simulink model "Vcu"  (R2020a)
settings: Solver=FixedStepDiscrete  StartTime=0.0  StopTime=10.0  FixedStep=ModelSimTime  RelTol=1e-3
PostLoadFcn:
  | , if any(exist('dsrtsu_mdlpostloadfcn', 'file') ~= 0), dsrtsu_mdlpostloadfcn('Execute', bdroot); end,
InitFcn:
  | , if any(exist('rtifpga_mdlclblib', 'file') ~= 0), rtifpga_mdlclblib('Init', bdroot); end,
undefined symbols (not defined in the file): rticanmm_blockfcn, rticanmm_initfcn, sigbuilder_block
libraries: rtimmsu_dsrtlib x5, commutil2 x1
(part 2 of 3)

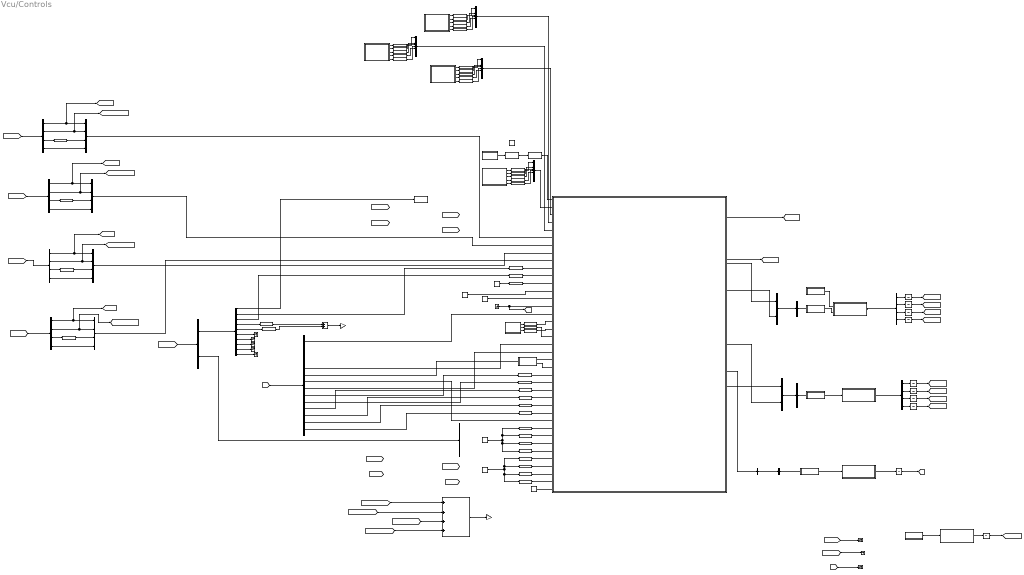
== system Vcu/Controls  ==
  Add : Sum  Inputs=++++
  Add1 : Sum  AccumDataTypeStr=double
  Bus Creator : BusCreator  Inputs=2
  Bus Creator1 : BusCreator  Inputs=2
  Bus Creator{7..10} (4 alike) : BusCreator  Inputs=11
  Bus Creator2 : BusCreator  Inputs=1
  Bus Creator{3..6} (4 alike) : BusCreator  Inputs=4  OutDataTypeStr=Bus: AmkActualValues2
  Bus Selector : BusSelector  OutputSignals=Inverter1FL,Inverter2FR  OutputAsBus=on
  Bus Selector1 : BusSelector  OutputSignals=AMK0_ActualValues1,AMK1_ActualValues1,AMK0_ActualValues2,AMK1_ActualValues2
  Bus Selector10 : BusSelector  OutputSignals=MotorLoopFluidTemp,InverterLoopFluidTemp,MotorLoopPressure,InverterLoopPressure
  Bus Selector11 : BusSelector  OutputSignals=ELP_StateInfo.ELP_BmsFault,ELP_StateInfo.ELP_ContactorK1,ELP_StateInfo.ELP_ContactorK2,ELP_StateInfo.ELP_ContactorK3,ELP_StateInfo.ELP_RelayFault,ELP_StateInfo.ELP_Flags_uint8,ELP_StateInfo.ELP_FltCodeStored_uint8,ELP_StateInfo.ELP_LevelFaultFlags,ELP_SOCInfo.ELP_SOC_pc,ELP_CurrentInfo.ELP_PackCurrent_A,ELP_CurrentInfo.ELP_ChargeCurrentMax_A,ELP_CurrentInfo.ELP_DischargeCurrentMax_A,ELP_VoltageInfo.ELP_PackVoltage_V,ELP_TemperatureInfo.ELP_PackAvgTemp_degC
  Bus Selector{4..6,12} (4 alike) : BusSelector  OutputSignals=AMK_TempMotor,AMK_TempInverter,AMK_ErrorInfo,AMK_TempIGBT
  Bus Selector2 : BusSelector  OutputSignals=AMK0_ActualValues1,AMK1_ActualValues1,AMK0_ActualValues2,AMK1_ActualValues2
  Bus Selector3 : BusSelector  OutputSignals=Inverter3RL,Inverter4RR  OutputAsBus=on
  Bus Selector7 : BusSelector  OutputSignals=contactor  OutputAsBus=on
  Bus Selector8 : BusSelector  OutputSignals=DriveButton,AcceleratorPedalPosition0,AcceleratorPedalPosition1,BrakePedalPosition0,BrakePedalPosition1,Apps0Status,Apps1Status,Bpps0Status,Bpps1Status,BspdFault
  Bus Selector9 : BusSelector  OutputSignals=PedalPositions,CoolingLoopsData
  Cast To Boolean{,1..22} (23 alike) : DataTypeConversion  OutDataTypeStr=boolean
  Constant : Constant
  Constant1 : Constant
  Constant2 : Constant  Value=20
  Constant3 : Constant  Value=20
  Constant4 : Constant  Value=20
  Constant6 : Constant  Value=100
  Constant7 : Constant  Value=0
  Data Type Conversion : DataTypeConversion  OutDataTypeStr=Enum: DRIVER_BUTTON
  Data Type Conversion{1..23} (23 alike) : DataTypeConversion  OutDataTypeStr=double
  Data Type Conversion24 : DataTypeConversion  OutDataTypeStr=Enum: DRIVER_BUTTON
  Data Type Conversion25 : DataTypeConversion  OutDataTypeStr=uint8
  Gain : Gain  Gain=1/4
  Gain1 : Gain  Gain=1/2  OutDataTypeStr=double
  Ground : Ground
  Model : ModelReference  ModelNameDialog=Controls.slx  SimulationMode=Normal  ModelReferenceVersion=1.57
  RTICANMM MainBlock : Subsystem  InitFcn=rticanmm_blockfcn('InitFcn', 'CANnedy', gcb)  ClipboardFcn=rticanmm_blockfcn('ClipboardFcn', 'CANnedy', gcb)  mask(RTICANMM){DSProperties=struct('RTI',struct('Version',uint32(1),'BlockType',struct('isSLSource',uint8(1),'isSLSink',uint8(1),'isHWSource',uint8(0),'isHWSink',uint8(0),'isSetup',uint8(0),'isInline',uint8(1),'isNonInline',uint8(0),'isInterrupt',uint8(0),'isChannelwise',uint8(0)),'IOBoardType','RTICANMM','UnitType','RTICANMM','Identifier','Mainblock','DialogType','SL','BlockSet','RTICANMM','SlaveProcessor','CAN')), CANMMProperties=struct('RTICANMMVersion','5.4','RTICANMMVersionIntern','5.4.737888.359837963','RTICANMMDate','02-May-2020','Settings','RTICANMM_MAIN_CAN_Amk1','UserTracePath','','ModelPath','C:\Users\harjo\Git\MACFormulaGit\MicroAutobox\microAutoboxModels\ControlsVcu','filesettings',struct('FileName','..\..\..\CAN_Databases\CAN_AMKInverter_1.dbc','IsRelative',1,'ClusterId',1,'ClusterList',{{'default'}},'destfolder',struct('Name','RTICANMM_FILES','Check',1),'buildfolder',struct('Name','.','Check',1),'onlyfreerawcapture',0,'overlapping2variant',0,'canfdsupport',0,'shortestJ2container',1),'onlyfreerawcapture',0,'Board',['CAN Type 1'],'BoardNum','1','ChannelNum','1','Variation','1','SetupId','Amk1','MARK',['30B141190671575CDE9C61D58C158C';'625D2D9E4FA6805ED198087D0F7A70';'291D995F13C69D1BB521FD81278AB5';'0D32706B1F9558B19EB16214799388';'2E4D033EB29162329D08EE38258F6F'],'date','08-Jul-2020','clock',['08.07.2020 00:50:18'],'recreate',0,'RTIVER','RTI1401','j1939',0,'TRC',struct('include',1),'rtsupport',struct('XMLFile','C:\Users\harjo\Git\MACFormulaGit\MicroAutobox\microAutoboxModels\ControlsVcu\RTICANMM_FILES\RTICANMM_MAIN_CAN_Amk1.xml','DBCXML',struct('Path','C:\Users\harjo\Git\MACFormulaGit\MicroAutobox\microAutoboxModels\ControlsVcu\RTICANMM_FILES\RTICANMM_MAIN_CAN_Amk1_dbc.xml','support',1,'Name','CAN_AMKInverter_1.dbc','Date',['23-Sep-2019 17:54:42'],'Type','standard','DBCSupport','ON'))), CANMMType=CANnedy, CANMMUserTraceMerged=off, CANMMUserTracePath=, CANMMChannelNum=1, CANMMBoardNum=1, CANMMDestFolder=RTICANMM_FILES, CANMMFolder=., CANMMSetupId=Amk1, CANMMsave2mat=['30B141190671575CDE9C61D58C158C';'625D2D9E4FA6805ED198087D0F7A70';'291D995F13C69D1BB521FD81278AB5';'0D32706B1F9558B19EB16214799388';'2E4D033EB29162329D08EE38258F6F'], CANMMName=CAN_Amk1, CANMMSettings=RTICANMM_MAIN_CAN_Amk1, CANMMIntermediateTag=RTICANMM_MAIN_CAN_Amk1_intermediate, CANMMsfcnname=RTICANMM_MAIN_CAN_Amk1}
      mask init:
      | rticanmm_initfcn(gcb, CANMMType, CANMMsfcnname)
      settings: AttributesFormatString=Amk1[CAN_Amk1]: DS1401_B1_C1_V1  CopyFcn=rticanmm_blockfcn('CopyFcn', 'CANnedy', gcb)  DeleteFcn=rticanmm_blockfcn('DeleteFcn', 'CANnedy', gcb)  ModelCloseFcn=rticanmm_blockfcn('ModelCloseFcn', 'CANnedy', gcb)  NameChangeFcn=rticanmm_blockfcn('NameChangeFcn', 'CANnedy', gcb)  OpenFcn=try, rticanmm_main_gui('create',gcb); ; catch,errordlg({lasterr, '','Please check your RTI installation.'},['Error: ' upper(bdroot)], 'replace'); end  MoveFcn=rticanmm_blockfcn('MoveFcn', 'CANnedy', gcb)
      mask Help: eval('rticanmm_quickstart(''create'', gcb);', 'disp(lasterr);')
      mask Display:
      | disp(sprintf('RTI CAN\nMultiMessage\nMainBlock'))
      | port_label('input', 1, 'Triggering')
      | port_label('input', 2, 'TX Data')
      | port_label('output', 1, 'RX Data')
  RTICANMM MainBlock1 : Subsystem  InitFcn=rticanmm_blockfcn('InitFcn', 'CANnedy', gcb)  ClipboardFcn=rticanmm_blockfcn('ClipboardFcn', 'CANnedy', gcb)  mask(RTICANMM){DSProperties=struct('RTI',struct('Version',uint32(1),'BlockType',struct('isSLSource',uint8(1),'isSLSink',uint8(1),'isHWSource',uint8(0),'isHWSink',uint8(0),'isSetup',uint8(0),'isInline',uint8(1),'isNonInline',uint8(0),'isInterrupt',uint8(0),'isChannelwise',uint8(0)),'IOBoardType','RTICANMM','UnitType','RTICANMM','Identifier','Mainblock','DialogType','SL','BlockSet','RTICANMM','SlaveProcessor','CAN')), CANMMProperties=struct('RTICANMMVersion','5.4','RTICANMMVersionIntern','5.4.737888.359837963','RTICANMMDate','02-May-2020','Settings','RTICANMM_MAIN_CAN_Amk2','UserTracePath','','ModelPath','C:\Users\harjo\Git\MACFormulaGit\MicroAutobox\microAutoboxModels\ControlsVcu','filesettings',struct('FileName','..\..\..\CAN_Databases\CAN_AMKInverter_2.dbc','IsRelative',1,'ClusterId',1,'ClusterList',{{'default'}},'destfolder',struct('Name','RTICANMM_FILES','Check',1),'buildfolder',struct('Name','.','Check',1),'onlyfreerawcapture',0,'overlapping2variant',0,'canfdsupport',0,'shortestJ2container',1),'onlyfreerawcapture',0,'Board',['CAN Type 1'],'BoardNum','1','ChannelNum','2','Variation','1','SetupId','Amk2','MARK',['23D358A6111267E79AAC03A71D3B3C';'8056A98F5AF9351F3E7CAA9A529355';'6A9E9F0BDFBC277DE5492F546A53C6';'5C5711521DDD45BA998B60BD2F425C';'4BA44A73C7F91456F57C068350BFE8'],'date','08-Jul-2020','clock',['08.07.2020 00:53:31'],'recreate',0,'RTIVER','RTI1401','j1939',0,'TRC',struct('include',1),'rtsupport',struct('XMLFile','C:\Users\harjo\Git\MACFormulaGit\MicroAutobox\microAutoboxModels\ControlsVcu\RTICANMM_FILES\RTICANMM_MAIN_CAN_Amk2.xml','DBCXML',struct('Path','C:\Users\harjo\Git\MACFormulaGit\MicroAutobox\microAutoboxModels\ControlsVcu\RTICANMM_FILES\RTICANMM_MAIN_CAN_Amk2_dbc.xml','support',1,'Name','CAN_AMKInverter_2.dbc','Date',['27-May-2019 19:06:45'],'Type','standard','DBCSupport','ON'))), CANMMType=CANnedy, CANMMUserTraceMerged=off, CANMMUserTracePath=, CANMMChannelNum=2, CANMMBoardNum=1, CANMMDestFolder=RTICANMM_FILES, CANMMFolder=., CANMMSetupId=Amk2, CANMMsave2mat=['23D358A6111267E79AAC03A71D3B3C';'8056A98F5AF9351F3E7CAA9A529355';'6A9E9F0BDFBC277DE5492F546A53C6';'5C5711521DDD45BA998B60BD2F425C';'4BA44A73C7F91456F57C068350BFE8'], CANMMName=CAN_Amk2, CANMMSettings=RTICANMM_MAIN_CAN_Amk2, CANMMIntermediateTag=RTICANMM_MAIN_CAN_Amk2_intermediate, CANMMsfcnname=RTICANMM_MAIN_CAN_Amk2}
      mask init:
      | rticanmm_initfcn(gcb, CANMMType, CANMMsfcnname)
      settings: AttributesFormatString=Amk2[CAN_Amk2]: DS1401_B1_C2_V1  CopyFcn=rticanmm_blockfcn('CopyFcn', 'CANnedy', gcb)  DeleteFcn=rticanmm_blockfcn('DeleteFcn', 'CANnedy', gcb)  ModelCloseFcn=rticanmm_blockfcn('ModelCloseFcn', 'CANnedy', gcb)  NameChangeFcn=rticanmm_blockfcn('NameChangeFcn', 'CANnedy', gcb)  OpenFcn=try, rticanmm_main_gui('create',gcb); ; catch,errordlg({lasterr, '','Please check your RTI installation.'},['Error: ' upper(bdroot)], 'replace'); end  MoveFcn=rticanmm_blockfcn('MoveFcn', 'CANnedy', gcb)
      mask Help: eval('rticanmm_quickstart(''create'', gcb);', 'disp(lasterr);')
      mask Display:
      | disp(sprintf('RTI CAN\nMultiMessage\nMainBlock'))
      | port_label('input', 1, 'TX Data')
      | port_label('output', 1, 'RX Data')
  RTICANMM MainBlock2 : Subsystem  InitFcn=rticanmm_blockfcn('InitFcn', 'CANnedy', gcb)  ClipboardFcn=rticanmm_blockfcn('ClipboardFcn', 'CANnedy', gcb)  mask(RTICANMM){DSProperties=struct('RTI',struct('Version',uint32(1),'BlockType',struct('isSLSource',uint8(1),'isSLSink',uint8(1),'isHWSource',uint8(0),'isHWSink',uint8(0),'isSetup',uint8(0),'isInline',uint8(1),'isNonInline',uint8(0),'isInterrupt',uint8(0),'isChannelwise',uint8(0)),'IOBoardType','RTICANMM','UnitType','RTICANMM','Identifier','Mainblock','DialogType','SL','BlockSet','RTICANMM','SlaveProcessor','CAN')), CANMMProperties=struct('RTICANMMVersion','5.4','RTICANMMVersionIntern','5.4.737888.359837963','RTICANMMDate','02-May-2020','Settings','RTICANMM_MAIN_CAN_Driver','UserTracePath','','ModelPath','C:\Users\harjo\Git\MACFormulaGit\MicroAutobox\microAutoboxModels\ControlsVcu','filesettings',struct('FileName','..\..\..\CAN_Databases\CAN_Driver.dbc','IsRelative',1,'ClusterId',1,'ClusterList',{{'default'}},'destfolder',struct('Name','RTICANMM_FILES','Check',1),'buildfolder',struct('Name','.','Check',1),'onlyfreerawcapture',0,'overlapping2variant',0,'canfdsupport',0,'shortestJ2container',1),'onlyfreerawcapture',0,'Board',['CAN Type 1'],'BoardNum','2','ChannelNum','2','Variation','1','SetupId','Driver','MARK',['1FBDB5055509519A3D88242C53EAF0';'0F3EA1466D2C01C48DAB8B5A544B5E';'51622B8FF557AF490620283A560302';'5C1A7E59B50D6A3AADA77BEDA3831B';'9E3A065D5DEB0173F6A7D3160A2573'],'date','08-Jul-2020','clock',['08.07.2020 00:52:33'],'recreate',0,'RTIVER','RTI1401','j1939',0,'TRC',struct('include',1),'rtsupport',struct('XMLFile','C:\Users\harjo\Git\MACFormulaGit\MicroAutobox\microAutoboxModels\ControlsVcu\RTICANMM_FILES\RTICANMM_MAIN_CAN_Driver.xml','DBCXML',struct('Path','C:\Users\harjo\Git\MACFormulaGit\MicroAutobox\microAutoboxModels\ControlsVcu\RTICANMM_FILES\RTICANMM_MAIN_CAN_Driver_dbc.xml','support',1,'Name','CAN_Driver.dbc','Date',['10-Jun-2020 08:59:56'],'Type','standard','DBCSupport','ON'))), CANMMType=CANnedy, CANMMUserTraceMerged=off, CANMMUserTracePath=, CANMMChannelNum=2, CANMMBoardNum=2, CANMMDestFolder=RTICANMM_FILES, CANMMFolder=., CANMMSetupId=Driver, CANMMsave2mat=['1FBDB5055509519A3D88242C53EAF0';'0F3EA1466D2C01C48DAB8B5A544B5E';'51622B8FF557AF490620283A560302';'5C1A7E59B50D6A3AADA77BEDA3831B';'9E3A065D5DEB0173F6A7D3160A2573'], CANMMName=CAN_Driver, CANMMSettings=RTICANMM_MAIN_CAN_Driver, CANMMIntermediateTag=RTICANMM_MAIN_CAN_Driver_intermediate, CANMMsfcnname=RTICANMM_MAIN_CAN_Driver}
      mask init:
      | rticanmm_initfcn(gcb, CANMMType, CANMMsfcnname)
      settings: AttributesFormatString=Driver[CAN_Driver]: DS1401_B2_C2_V1  CopyFcn=rticanmm_blockfcn('CopyFcn', 'CANnedy', gcb)  DeleteFcn=rticanmm_blockfcn('DeleteFcn', 'CANnedy', gcb)  ModelCloseFcn=rticanmm_blockfcn('ModelCloseFcn', 'CANnedy', gcb)  NameChangeFcn=rticanmm_blockfcn('NameChangeFcn', 'CANnedy', gcb)  OpenFcn=try, rticanmm_main_gui('create',gcb); ; catch,errordlg({lasterr, '','Please check your RTI installation.'},['Error: ' upper(bdroot)], 'replace'); end  MoveFcn=rticanmm_blockfcn('MoveFcn', 'CANnedy', gcb)
      mask Help: eval('rticanmm_quickstart(''create'', gcb);', 'disp(lasterr);')
      mask Display:
      | disp(sprintf('RTI CAN\nMultiMessage\nMainBlock'))
      | port_label('input', 1, 'TX Data')
      | port_label('output', 1, 'RX Data')
  RTICANMM MainBlock3 : Subsystem  InitFcn=rticanmm_blockfcn('InitFcn', 'CANnedy', gcb)  ClipboardFcn=rticanmm_blockfcn('ClipboardFcn', 'CANnedy', gcb)  mask(RTICANMM){DSProperties=struct('RTI',struct('Version',uint32(1),'BlockType',struct('isSLSource',uint8(1),'isSLSink',uint8(1),'isHWSource',uint8(0),'isHWSink',uint8(0),'isSetup',uint8(0),'isInline',uint8(1),'isNonInline',uint8(0),'isInterrupt',uint8(0),'isChannelwise',uint8(0)),'IOBoardType','RTICANMM','UnitType','RTICANMM','Identifier','Mainblock','DialogType','SL','BlockSet','RTICANMM','SlaveProcessor','CAN')), CANMMProperties=struct('RTICANMMVersion','5.4','RTICANMMVersionIntern','5.4.737888.359837963','RTICANMMDate','02-May-2020','Settings','RTICANMM_MAIN_CAN_Ams','UserTracePath','','ModelPath','C:\Users\harjo\Git\MACFormulaGit\MicroAutobox\microAutoboxModels\ControlsVcu','filesettings',struct('FileName','..\..\..\CAN_Databases\CAN_ESS.dbc','IsRelative',1,'ClusterId',1,'ClusterList',{{'default'}},'destfolder',struct('Name','RTICANMM_FILES','Check',1),'buildfolder',struct('Name','.','Check',1),'onlyfreerawcapture',0,'overlapping2variant',0,'canfdsupport',0,'shortestJ2container',1),'onlyfreerawcapture',0,'Board',['CAN Type 1'],'BoardNum','2','ChannelNum','1','Variation','1','SetupId','Ams','MARK',['6F3BE71B63DA823D8A5738BC21B280';'7BE5148685F49B17D08A9A02A74A0A';'4309FE7EF19F1E2F6299CF556E3CA3';'29B8269B22424F2A37A5AD46A8EF39';'04763123DE2E10B216A1C66D7AE016'],'date','08-Jul-2020','clock',['08.07.2020 00:51:39'],'recreate',0,'RTIVER','RTI1401','j1939',0,'TRC',struct('include',1),'rtsupport',struct('XMLFile','C:\Users\harjo\Git\MACFormulaGit\MicroAutobox\microAutoboxModels\ControlsVcu\RTICANMM_FILES\RTICANMM_MAIN_CAN_Ams.xml','DBCXML',struct('Path','C:\Users\harjo\Git\MACFormulaGit\MicroAutobox\microAutoboxModels\ControlsVcu\RTICANMM_FILES\RTICANMM_MAIN_CAN_Ams_dbc.xml','support',1,'Name','CAN_ESS.dbc','Date',['27-May-2019 19:33:31'],'Type','standard','DBCSupport','ON'))), CANMMType=CANnedy, CANMMUserTraceMerged=off, CANMMUserTracePath=, CANMMChannelNum=1, CANMMBoardNum=2, CANMMDestFolder=RTICANMM_FILES, CANMMFolder=., CANMMSetupId=Ams, CANMMsave2mat=['6F3BE71B63DA823D8A5738BC21B280';'7BE5148685F49B17D08A9A02A74A0A';'4309FE7EF19F1E2F6299CF556E3CA3';'29B8269B22424F2A37A5AD46A8EF39';'04763123DE2E10B216A1C66D7AE016'], CANMMName=CAN_Ams, CANMMSettings=RTICANMM_MAIN_CAN_Ams, CANMMIntermediateTag=RTICANMM_MAIN_CAN_Ams_intermediate, CANMMsfcnname=RTICANMM_MAIN_CAN_Ams}
      mask init:
      | rticanmm_initfcn(gcb, CANMMType, CANMMsfcnname)
      settings: AttributesFormatString=Ams[CAN_Ams]: DS1401_B2_C1_V1  CopyFcn=rticanmm_blockfcn('CopyFcn', 'CANnedy', gcb)  DeleteFcn=rticanmm_blockfcn('DeleteFcn', 'CANnedy', gcb)  ModelCloseFcn=rticanmm_blockfcn('ModelCloseFcn', 'CANnedy', gcb)  NameChangeFcn=rticanmm_blockfcn('NameChangeFcn', 'CANnedy', gcb)  OpenFcn=try, rticanmm_main_gui('create',gcb); ; catch,errordlg({lasterr, '','Please check your RTI installation.'},['Error: ' upper(bdroot)], 'replace'); end  MoveFcn=rticanmm_blockfcn('MoveFcn', 'CANnedy', gcb)
      mask Help: eval('rticanmm_quickstart(''create'', gcb);', 'disp(lasterr);')
      mask Display:
      | disp(sprintf('RTI CAN\nMultiMessage\nMainBlock'))
      | port_label('input', 1, 'TX Data')
      | port_label('output', 1, 'RX Data')
  Signal Builder : Subsystem  Tag=STV Subsys  LoadFcn=sigbuilder_block('load');  StartFcn=sigbuilder_block('start');  StopFcn=sigbuilder_block('stop');  ClipboardFcn=sigbuilder_block('clipboard');  mask(Sigbuilder block){tuvar=[0:10]}
      mask help: Simulink:masks:SigbuilderBlock_MD
      mask init:
      | if ~strcmp(get_param(bdroot(gcbh),'SimulationStatus'),'stopped') tuvar = sigbuilder_block('maskInit'); end
      settings: CopyFcn=sigbuilder_block('copy');  DeleteFcn=sigbuilder_block('delete');  ModelCloseFcn=sigbuilder_block('modelClose');  PreSaveFcn=sigbuilder_block('preSave');  PauseFcn=sigbuilder_block('pause');  ContinueFcn=sigbuilder_block('continue');  NameChangeFcn=sigbuilder_block('namechange');  OpenFcn=sigbuilder_block('open',[7.5 294 951 452.25 ]);  CloseFcn=sigbuilder_block('close');
      mask Display: plot(0, 0, 100, 100,[2, 2, 32, 32, 2], [68, 8, 8, 68, 68],[32, 2], [38, 38], [32, 19, 2],[53, 60, 44], [32, 17, 17, 2],[16, 16, 31, 31]);txt = getActiveGroup(gcbh);text(2, 100, txt,'verticalAlignment', 'top');
  Signal Builder1 : Subsystem  Tag=STV Subsys  LoadFcn=sigbuilder_block('load');  StartFcn=sigbuilder_block('start');  StopFcn=sigbuilder_block('stop');  ClipboardFcn=sigbuilder_block('clipboard');  mask(Sigbuilder block){tuvar=[0:10]}
      mask help: Simulink:masks:SigbuilderBlock_MD
      mask init:
      | if ~strcmp(get_param(bdroot(gcbh),'SimulationStatus'),'stopped') tuvar = sigbuilder_block('maskInit'); end
      settings: CopyFcn=sigbuilder_block('copy');  DeleteFcn=sigbuilder_block('delete');  ModelCloseFcn=sigbuilder_block('modelClose');  PreSaveFcn=sigbuilder_block('preSave');  PauseFcn=sigbuilder_block('pause');  ContinueFcn=sigbuilder_block('continue');  NameChangeFcn=sigbuilder_block('namechange');  OpenFcn=sigbuilder_block('open',[4.8 22.8 950.4 430.8 ]);  CloseFcn=sigbuilder_block('close');
      mask Display: plot(0, 0, 100, 100,[2, 2, 32, 32, 2], [68, 8, 8, 68, 68],[32, 2], [38, 38], [32, 19, 2],[53, 60, 44], [32, 17, 17, 2],[16, 16, 31, 31]);txt = getActiveGroup(gcbh);text(2, 100, txt,'verticalAlignment', 'top');
  Signal Builder2 : Subsystem  Tag=STV Subsys  LoadFcn=sigbuilder_block('load');  StartFcn=sigbuilder_block('start');  StopFcn=sigbuilder_block('stop');  ClipboardFcn=sigbuilder_block('clipboard');  mask(Sigbuilder block){tuvar=[0:10]}
      mask help: Simulink:masks:SigbuilderBlock_MD
      mask init:
      | if ~strcmp(get_param(bdroot(gcbh),'SimulationStatus'),'stopped') tuvar = sigbuilder_block('maskInit'); end
      settings: CopyFcn=sigbuilder_block('copy');  DeleteFcn=sigbuilder_block('delete');  ModelCloseFcn=sigbuilder_block('modelClose');  PreSaveFcn=sigbuilder_block('preSave');  PauseFcn=sigbuilder_block('pause');  ContinueFcn=sigbuilder_block('continue');  NameChangeFcn=sigbuilder_block('namechange');  OpenFcn=sigbuilder_block('open',[4.8 66.3 950.4 417.3 ]);  CloseFcn=sigbuilder_block('close');
      mask Display: plot(0, 0, 100, 100,[2, 2, 32, 32, 2], [68, 8, 8, 68, 68],[32, 2], [38, 38], [32, 19, 2],[53, 60, 44], [32, 17, 17, 2],[16, 16, 31, 31]);txt = getActiveGroup(gcbh);text(2, 100, txt,'verticalAlignment', 'top');
  Signal Builder3 : Subsystem  Tag=STV Subsys  LoadFcn=sigbuilder_block('load');  StartFcn=sigbuilder_block('start');  StopFcn=sigbuilder_block('stop');  ClipboardFcn=sigbuilder_block('clipboard');  mask(Sigbuilder block){tuvar=[0:10]}
      mask help: Simulink:masks:SigbuilderBlock_MD
      mask init:
      | if ~strcmp(get_param(bdroot(gcbh),'SimulationStatus'),'stopped') tuvar = sigbuilder_block('maskInit'); end
      settings: CopyFcn=sigbuilder_block('copy');  DeleteFcn=sigbuilder_block('delete');  ModelCloseFcn=sigbuilder_block('modelClose');  PreSaveFcn=sigbuilder_block('preSave');  PauseFcn=sigbuilder_block('pause');  ContinueFcn=sigbuilder_block('continue');  NameChangeFcn=sigbuilder_block('namechange');  OpenFcn=sigbuilder_block('open',[4.8 66.3 950.4 417.3 ]);  CloseFcn=sigbuilder_block('close');
      mask Display: plot(0, 0, 100, 100,[2, 2, 32, 32, 2], [68, 8, 8, 68, 68],[32, 2], [38, 38], [32, 19, 2],[53, 60, 44], [32, 17, 17, 2],[16, 16, 31, 31]);txt = getActiveGroup(gcbh);text(2, 100, txt,'verticalAlignment', 'top');
  Signal Builder4 : Subsystem  Tag=STV Subsys  LoadFcn=sigbuilder_block('load');  StartFcn=sigbuilder_block('start');  StopFcn=sigbuilder_block('stop');  ClipboardFcn=sigbuilder_block('clipboard');  mask(Sigbuilder block){tuvar=[0:10]}
      mask help: Simulink:masks:SigbuilderBlock_MD
      mask init:
      | if ~strcmp(get_param(bdroot(gcbh),'SimulationStatus'),'stopped') tuvar = sigbuilder_block('maskInit'); end
      settings: CopyFcn=sigbuilder_block('copy');  DeleteFcn=sigbuilder_block('delete');  ModelCloseFcn=sigbuilder_block('modelClose');  PreSaveFcn=sigbuilder_block('preSave');  PauseFcn=sigbuilder_block('pause');  ContinueFcn=sigbuilder_block('continue');  NameChangeFcn=sigbuilder_block('namechange');  OpenFcn=sigbuilder_block('open',[4.8 66.3 950.4 417.3 ]);  CloseFcn=sigbuilder_block('close');
      mask Display: plot(0, 0, 100, 100,[2, 2, 32, 32, 2], [68, 8, 8, 68, 68],[32, 2], [38, 38], [32, 19, 2],[53, 60, 44], [32, 17, 17, 2],[16, 16, 31, 31]);txt = getActiveGroup(gcbh);text(2, 100, txt,'verticalAlignment', 'top');
  Signal Builder5 : Subsystem  Tag=STV Subsys  LoadFcn=sigbuilder_block('load');  StartFcn=sigbuilder_block('start');  StopFcn=sigbuilder_block('stop');  ClipboardFcn=sigbuilder_block('clipboard');  mask(Sigbuilder block){tuvar=[0:10]}
      mask help: Simulink:masks:SigbuilderBlock_MD
      mask init:
      | if ~strcmp(get_param(bdroot(gcbh),'SimulationStatus'),'stopped') tuvar = sigbuilder_block('maskInit'); end
      settings: CopyFcn=sigbuilder_block('copy');  DeleteFcn=sigbuilder_block('delete');  ModelCloseFcn=sigbuilder_block('modelClose');  PreSaveFcn=sigbuilder_block('preSave');  PauseFcn=sigbuilder_block('pause');  ContinueFcn=sigbuilder_block('continue');  NameChangeFcn=sigbuilder_block('namechange');  OpenFcn=sigbuilder_block('open',[405 118.5 550.2 365.1 ]);  CloseFcn=sigbuilder_block('close');
      mask Display: plot(0, 0, 100, 100,[2, 2, 32, 32, 2], [68, 8, 8, 68, 68],[32, 2], [38, 38], [32, 19, 2],[53, 60, 44], [32, 17, 17, 2],[16, 16, 31, 31]);txt = getActiveGroup(gcbh);text(2, 100, txt,'verticalAlignment', 'top');
  Subsystem : Subsystem
  Terminator{1..3,5..9} (8 alike) : Terminator
  Triggering2RTICANMM MainBlock : Subsystem
      mask Display: disp('Triggering\nto RTICANMM')
  Unit Delay{,1..5,7..9,13} (10 alike) : UnitDelay  SampleTime=-1  HasFrameUpgradeWarning=on
  User2RTICANMM MainBlock : Subsystem
      mask Display: disp('Mapping\nto RTICANMM')
  User2RTICANMM MainBlock1 : Subsystem
      mask Display: disp('Mapping\nto RTICANMM')
  User2RTICANMM MainBlock2 : Subsystem
      mask Display: disp('Mapping\nto RTICANMM')
  User2RTICANMM MainBlock3 : Subsystem
      mask Display: disp('Mapping\nto RTICANMM')
  wires:
  User2RTICANMM MainBlock1/1(out) -> RTICANMM MainBlock1/1(TXData)
  Model/3 -> Bus Creator/1  "Inverter1FL"
  Bus Selector2/1 -> Unit Delay1/1  "<AMK0_ActualValues1>"
  Bus Creator1/1 -> Bus Selector3/1  "Amk2"
  User2RTICANMM MainBlock/1(out) -> RTICANMM MainBlock/2(TXData)
  Model/4 -> Bus Creator/2  "Inverter2FR"
  Bus Creator/1 -> Bus Selector/1  "Amk1"
  Bus Selector2/3 -> Unit Delay8/1  "<AMK0_ActualValues2>"
  Model/6 -> Bus Creator1/2  "Inverter4RR"
  Bus Selector1/4 -> Unit Delay5/1  "<AMK1_ActualValues2>"
  Bus Selector1/2 -> Unit Delay4/1  "<AMK1_ActualValues1>"
  Bus Selector1/3 -> Unit Delay13/1  "<AMK0_ActualValues2>"
  Bus Selector2/4 -> Unit Delay9/1  "<AMK1_ActualValues2>"
  Model/5 -> Bus Creator1/1  "Inverter3RL"
  Bus Selector2/2 -> Unit Delay7/1  "<AMK1_ActualValues1>"
  Bus Selector1/1 -> Unit Delay/1  "<AMK0_ActualValues1>"
  Bus Selector9/2 -> Bus Selector10/1  "<CoolingLoopsData>"
  [AMS] -> Bus Selector11/1
  Bus Selector11/1 -> Model/16  "<ELP_BmsFault>"
  Add1/1 -> Gain1/1
  [InverterColdPlateTempFR] -> Add/2
  [DriverRx] -> Bus Selector9/1
  Bus Selector9/1 -> Bus Selector8/1  "<PedalPositions>"
  User2RTICANMM MainBlock2/1(out) -> RTICANMM MainBlock2/1(TXData)
  [InverterColdPlateTempRR] -> Add/4
  RTICANMM MainBlock2/1(RX_Data) -> Unit Delay3/1
  Bus Selector8/3 -> Data Type Conversion13/1  "<AcceleratorPedalPosition1>"
  Bus Selector8/4 -> Data Type Conversion14/1  "<BrakePedalPosition0>"
  Bus Selector8/5 -> Data Type Conversion15/1  "<BrakePedalPosition1>"
  Add/1 -> Gain/1
  Bus Selector3/1 -> User2RTICANMM MainBlock1/1(in)
  Bus Selector8/1 -> Data Type Conversion/1  "<DriveButton>"
  Bus Selector8/2 -> Data Type Conversion12/1  "<AcceleratorPedalPosition0>"
  User2RTICANMM MainBlock3/1(out) -> RTICANMM MainBlock3/1(TXData)
  [InverterColdPlateTempFL] -> Add/1
  [InverterColdPlateTempRL] -> Add/3
  RTICANMM MainBlock3/1(RX_Data) -> Unit Delay2/1
  [VehicleStatus] -> Terminator1/1
  Subsystem/2(LLIM) -> Model/23
  Bus Selector11/7 -> Model/30  "<ELP_FltCodeStored_uint8>"
  Data Type Conversion4/1 -> Model/33
  Data Type Conversion6/1 -> Model/26
  Bus Selector11/11 -> Data Type Conversion6/1  "<ELP_ChargeCurrentMax_A>"
  Bus Selector11/6 -> Subsystem/1(AmsState)  "<ELP_Flags_uint8>"
  Bus Selector11/5 -> Model/20  "<ELP_RelayFault>"
  Bus Selector11/12 -> Data Type Conversion7/1  "<ELP_DischargeCurrentMax_A>"
  [RTDS_CAN] -> Terminator2/1
  Constant1/1 -> Model/14
  Data Type Conversion3/1 -> Model/32
  Subsystem/1(HLIM) -> Model/22
  Bus Selector11/14 -> Data Type Conversion11/1  "<ELP_PackAvgTemp_degC>"
  [Speed] -> Terminator3/1
  Bus Selector11/8 -> Model/21  "<ELP_LevelFaultFlags>"
  Bus Selector11/10 -> Data Type Conversion8/1  "<ELP_PackCurrent_A>"
  Model/1 -> [VehicleStatus]
  Model/2 -> [RTDS_CAN]
  Data Type Conversion1/1 -> Model/12
  Data Type Conversion2/1 -> Model/31
  Data Type Conversion5/1 -> Model/34
  Data Type Conversion7/1 -> Model/27
  Bus Selector11/13 -> Data Type Conversion10/1  "<ELP_PackVoltage_V>"
  Constant/1 -> Model/13
  Ground/1 -> [Speed], Model/15
  Bus Selector8/10 -> Terminator9/1  "<BspdFault>"
  Data Type Conversion12/1 -> Model/10
  Data Type Conversion8/1 -> Model/25
  Data Type Conversion11/1 -> Model/29
  Bus Selector8/6 -> Terminator5/1  "<Apps0Status>"
  Bus Selector8/8 -> Terminator7/1  "<Bpps0Status>"
  Bus Selector8/7 -> Terminator6/1  "<Apps1Status>"
  Data Type Conversion10/1 -> Model/28
  Bus Selector11/9 -> Data Type Conversion9/1  "<ELP_SOC_pc>"
  Unit Delay2/1 -> [AMS]
  Unit Delay3/1 -> [DriverRx]
  Data Type Conversion17/1 -> Model/35
  Bus Selector8/9 -> Terminator8/1  "<Bpps1Status>"
  Model/7 -> Bus Creator2/1  "contactor"
  RTICANMM MainBlock1/1(RX_Data) -> Bus Selector2/1
  Data Type Conversion16/1 -> Model/36
  Unit Delay/1 -> [AmkAv1FL]
  Data Type Conversion15/1 -> Add1/2
  Data Type Conversion14/1 -> Add1/1
  Unit Delay1/1 -> [AmkAv1RL]
  Unit Delay4/1 -> [AmkAv1FR]
  RTICANMM MainBlock/1(RX_Data) -> Bus Selector1/1
  Unit Delay7/1 -> [AmkAv1RR]
  Data Type Conversion18/1 -> Model/37
  Bus Creator4/1 -> Model/8
  Data Type Conversion13/1 -> Model/11
  Data Type Conversion19/1 -> Model/38
  Unit Delay8/1 -> [AmkAv2RL]
  Data Type Conversion9/1 -> Model/24
  [AmkAv2FR] -> Bus Selector4/1
  Bus Selector12/2 -> [InverterColdPlateTempRR], Bus Creator5/2  "<AMK_TempInverter>"
  Data Type Conversion21/1 -> Bus Creator4/3  "AMK_ErrorInfo"
  Data Type Conversion22/1 -> Bus Creator5/3  "AMK_ErrorInfo"
  Bus Creator5/1 -> Model/9
  Unit Delay9/1 -> [AmkAv2RR]
  Bus Selector4/3 -> Data Type Conversion20/1  "<AMK_ErrorInfo>"
  Data Type Conversion20/1 -> Bus Creator3/3  "AMK_ErrorInfo"
  Bus Selector5/3 -> Data Type Conversion21/1  "<AMK_ErrorInfo>"
  Bus Selector5/2 -> [InverterColdPlateTempRL], Bus Creator4/2  "<AMK_TempInverter>"
  Bus Selector12/3 -> Data Type Conversion22/1  "<AMK_ErrorInfo>"
  Bus Selector4/2 -> [InverterColdPlateTempFR], Bus Creator3/2  "<AMK_TempInverter>"
  Bus Selector5/1 -> [MotorTempRL], Bus Creator4/1  "<AMK_TempMotor>"
  Bus Selector5/4 -> Bus Creator4/4  "<AMK_TempIGBT>"
  Bus Selector12/4 -> Bus Creator5/4  "<AMK_TempIGBT>"
  Bus Selector4/4 -> Bus Creator3/4  "<AMK_TempIGBT>"
  Bus Selector6/2 -> [InverterColdPlateTempFL], Bus Creator6/2  "<AMK_TempInverter>"
  Bus Selector6/3 -> Data Type Conversion23/1  "<AMK_ErrorInfo>"
  Bus Selector4/1 -> [MotorTempFR], Bus Creator3/1  "<AMK_TempMotor>"
  [AmkAv2RR] -> Bus Selector12/1
  [AmkAv2RL] -> Bus Selector5/1
  Unit Delay5/1 -> [AmkAv2FR]
  Data Type Conversion23/1 -> Bus Creator6/3  "AMK_ErrorInfo"
  Bus Selector6/1 -> [MotorTempFL], Bus Creator6/1  "<AMK_TempMotor>"
  [AmkAv2FL] -> Bus Selector6/1
  Bus Selector6/4 -> Bus Creator6/4  "<AMK_TempIGBT>"
  Bus Creator6/1 -> Model/6
  Unit Delay13/1 -> [AmkAv2FL]
  Bus Selector12/1 -> [MotorTempRR], Bus Creator5/1  "<AMK_TempMotor>"
  Bus Creator3/1 -> Model/7
  Triggering2RTICANMM MainBlock/1(out) -> RTICANMM MainBlock/1(Triggering)
  Bus Selector/1 -> User2RTICANMM MainBlock/1(in)
  Bus Creator2/1 -> Bus Selector7/1
  Bus Selector7/1 -> User2RTICANMM MainBlock3/1(in)
  Constant2/1 -> Data Type Conversion19/1, Data Type Conversion18/1, Data Type Conversion16/1, Data Type Conversion17/1
  Constant3/1 -> Data Type Conversion3/1, Data Type Conversion2/1, Data Type Conversion4/1, Data Type Conversion5/1
  Constant4/1 -> Model/39
  Constant6/1 -> Data Type Conversion1/1
  Signal Builder/1(AMK_bSystemReady) -> Cast To Boolean/1
  Signal Builder/2(AMK_bDcOn) -> Cast To Boolean1/1
  Signal Builder/3(AMK_bQuitDcON) -> Cast To Boolean2/1
  Signal Builder/4(AMK_bInverterOn) -> Cast To Boolean3/1
  Signal Builder/5(AMK_bQuitInverterOn) -> Cast To Boolean4/1
  Cast To Boolean/1 -> Bus Creator7/1
  Cast To Boolean2/1 -> Bus Creator7/4
  Cast To Boolean1/1 -> Bus Creator7/5
  Cast To Boolean4/1 -> Bus Creator7/6
  Cast To Boolean3/1 -> Bus Creator7/7
  Signal Builder1/1(K1) -> Cast To Boolean5/1
  Signal Builder1/2(K3) -> Cast To Boolean6/1
  Signal Builder1/3(K2) -> Cast To Boolean7/1
  Cast To Boolean7/1 -> Model/18
  Cast To Boolean6/1 -> Model/19
  Cast To Boolean5/1 -> Model/17
  Data Type Conversion24/1 -> Model/1
  Bus Creator7/1 -> Model/2
  Cast To Boolean8/1 -> Bus Creator8/1
  Signal Builder2/5(AMK_bQuitInverterOn) -> Cast To Boolean12/1
  Cast To Boolean10/1 -> Bus Creator8/4
  Cast To Boolean12/1 -> Bus Creator8/6
  Cast To Boolean9/1 -> Bus Creator8/5
  Signal Builder2/2(AMK_bDcOn) -> Cast To Boolean9/1
  Signal Builder2/4(AMK_bInverterOn) -> Cast To Boolean11/1
  Signal Builder2/3(AMK_bQuitDcON) -> Cast To Boolean10/1
  Signal Builder2/1(AMK_bSystemReady) -> Cast To Boolean8/1
  Cast To Boolean11/1 -> Bus Creator8/7
  Bus Creator8/1 -> Model/3
  Cast To Boolean13/1 -> Bus Creator9/1
  Signal Builder3/5(AMK_bQuitInverterOn) -> Cast To Boolean17/1
  Cast To Boolean15/1 -> Bus Creator9/4
  Cast To Boolean17/1 -> Bus Creator9/6
  Cast To Boolean14/1 -> Bus Creator9/5
  Signal Builder3/2(AMK_bDcOn) -> Cast To Boolean14/1
  Signal Builder3/4(AMK_bInverterOn) -> Cast To Boolean16/1
  Signal Builder3/3(AMK_bQuitDcON) -> Cast To Boolean15/1
  Signal Builder3/1(AMK_bSystemReady) -> Cast To Boolean13/1
  Cast To Boolean16/1 -> Bus Creator9/7
  Bus Creator9/1 -> Model/4
  Cast To Boolean18/1 -> Bus Creator10/1
  Signal Builder4/5(AMK_bQuitInverterOn) -> Cast To Boolean22/1
  Cast To Boolean20/1 -> Bus Creator10/4
  Cast To Boolean22/1 -> Bus Creator10/6
  Cast To Boolean19/1 -> Bus Creator10/5
  Signal Builder4/2(AMK_bDcOn) -> Cast To Boolean19/1
  Signal Builder4/4(AMK_bInverterOn) -> Cast To Boolean21/1
  Signal Builder4/3(AMK_bQuitDcON) -> Cast To Boolean20/1
  Signal Builder4/1(AMK_bSystemReady) -> Cast To Boolean18/1
  Cast To Boolean21/1 -> Bus Creator10/7
  Bus Creator10/1 -> Model/5
  Signal Builder5/1(Driver Button) -> Data Type Conversion25/1
  Data Type Conversion25/1 -> Data Type Conversion24/1

== system Vcu/RTICANMM ControllerSetup ==
  VariationInput : Inport
  Reset : Inport  Port=2
  ModelClose : Subsystem  mask(RTICANMMModelClose){}
  RTICANMMCHANNEL_TLC : S-Function  FunctionName=rticanmm_tlc_adv  Parameters=1401,1,1,0,500,11143421  SFunctionDeploymentMode=off  EnableBusSupport=off  mask(RTICANMMCHANNEL_TLC){}
  Variation_DTC : DataTypeConversion  SaturateOnIntegerOverflow=on  RndMeth=Zero
  sfcn : S-Function  InitFcn=rticanmm_initfcn(gcb, 'SFCNs')  FunctionName=RTICANMM_SETUP_Amk1  SFunctionDeploymentMode=off  EnableBusSupport=off
      mask init:
      | rticanmm_initfcn(gcb, 'SFCNs')
  wires:
  Reset/1 -> sfcn/2
  VariationInput/1 -> Variation_DTC/1
  Variation_DTC/1 -> sfcn/1

== system Vcu/RTICANMM ControllerSetup1 ==
  VariationInput : Inport
  Reset : Inport  Port=2
  ModelClose : Subsystem  mask(RTICANMMModelClose){}
  RTICANMMCHANNEL_TLC : S-Function  FunctionName=rticanmm_tlc_adv  Parameters=1401,1,2,0,500,11243421  SFunctionDeploymentMode=off  EnableBusSupport=off  mask(RTICANMMCHANNEL_TLC){}
  Variation_DTC : DataTypeConversion  SaturateOnIntegerOverflow=on  RndMeth=Zero
  sfcn : S-Function  InitFcn=rticanmm_initfcn(gcb, 'SFCNs')  FunctionName=RTICANMM_SETUP_Amk2  SFunctionDeploymentMode=off  EnableBusSupport=off
      mask init:
      | rticanmm_initfcn(gcb, 'SFCNs')
  wires:
  Reset/1 -> sfcn/2
  VariationInput/1 -> Variation_DTC/1
  Variation_DTC/1 -> sfcn/1

== system Vcu/RTICANMM ControllerSetup2 ==
  VariationInput : Inport
  Reset : Inport  Port=2
  ModelClose : Subsystem  mask(RTICANMMModelClose){}
  RTICANMMCHANNEL_TLC : S-Function  FunctionName=rticanmm_tlc_adv  Parameters=1401,2,1,0,500,12143421  SFunctionDeploymentMode=off  EnableBusSupport=off  mask(RTICANMMCHANNEL_TLC){}
  Variation_DTC : DataTypeConversion  SaturateOnIntegerOverflow=on  RndMeth=Zero
  sfcn : S-Function  InitFcn=rticanmm_initfcn(gcb, 'SFCNs')  FunctionName=RTICANMM_SETUP_Ams  SFunctionDeploymentMode=off  EnableBusSupport=off
      mask init:
      | rticanmm_initfcn(gcb, 'SFCNs')
  wires:
  Reset/1 -> sfcn/2
  VariationInput/1 -> Variation_DTC/1
  Variation_DTC/1 -> sfcn/1

== system Vcu/RTICANMM ControllerSetup3 ==
  VariationInput : Inport
  Reset : Inport  Port=2
  ModelClose : Subsystem  mask(RTICANMMModelClose){}
  RTICANMMCHANNEL_TLC : S-Function  FunctionName=rticanmm_tlc_adv  Parameters=1401,2,2,0,500,12243421  SFunctionDeploymentMode=off  EnableBusSupport=off  mask(RTICANMMCHANNEL_TLC){}
  Variation_DTC : DataTypeConversion  SaturateOnIntegerOverflow=on  RndMeth=Zero
  sfcn : S-Function  InitFcn=rticanmm_initfcn(gcb, 'SFCNs')  FunctionName=RTICANMM_SETUP_Driver  SFunctionDeploymentMode=off  EnableBusSupport=off
      mask init:
      | rticanmm_initfcn(gcb, 'SFCNs')
  wires:
  Reset/1 -> sfcn/2
  VariationInput/1 -> Variation_DTC/1
  Variation_DTC/1 -> sfcn/1

== system Vcu/RTICANMM GeneralSetup ==
  Constant : Constant
  ModelClose : Subsystem  mask(RTICANMMModelClose){}
  TRC Exclusion : rtimmsu_dsrtlib/TRC Exclusion
  Terminator : Terminator
  wires:
  Constant/1 -> Terminator/1

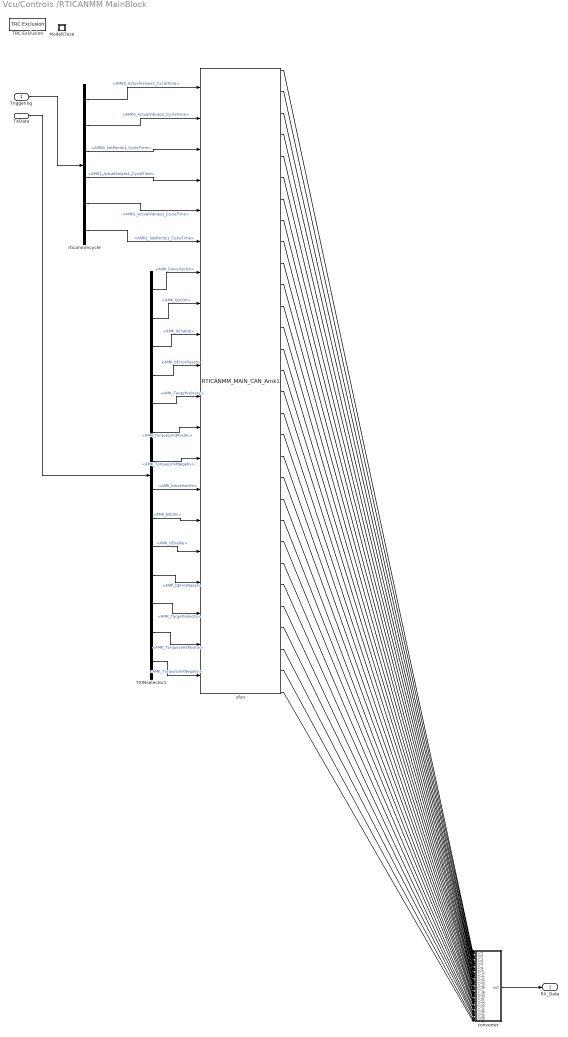
== system Vcu/Controls /RTICANMM MainBlock ==
  Triggering : Inport
  TXData : Inport  Port=2
  ModelClose : Subsystem  mask(RTICANMMModelClose){}
  TRC Exclusion : rtimmsu_dsrtlib/TRC Exclusion
  TXINselector1 : BusSelector  OutputSignals=AMK0_SetPoints1.AMK_bInverterOn,AMK0_SetPoints1.AMK_bDcOn,AMK0_SetPoints1.AMK_bEnable,AMK0_SetPoints1.AMK_bErrorReset,AMK0_SetPoints1.AMK_TargetVelocity,AMK0_SetPoints1.AMK_TorqueLimitPositiv,AMK0_SetPoints1.AMK_TorqueLimitNegativ,AMK1_SetPoints1.AMK_bInverterOn,AMK1_SetPoints1.AMK_bDcOn,AMK1_SetPoints1.AMK_bEnable,AMK1_SetPoints1.AMK_bErrorReset,AMK1_SetPoints1.AMK_TargetVelocity,AMK1_SetPoints1.AMK_TorqueLimitPositiv,AMK1_SetPoints1.AMK_TorqueLimitNegativ
  converter : Subsystem  mask(CANnedyVector2Bus){}
      mask help: Do not change.
      mask Display: disp('Vector to\nBus')
  rticanmmcycle : BusSelector  OutputSignals=AMK0_ActualValues1.AMK0_ActualValues1_CycleTime,AMK0_ActualValues2.AMK0_ActualValues2_CycleTime,AMK0_SetPoints1.AMK0_SetPoints1_CycleTime,AMK1_ActualValues1.AMK1_ActualValues1_CycleTime,AMK1_ActualValues2.AMK1_ActualValues2_CycleTime,AMK1_SetPoints1.AMK1_SetPoints1_CycleTime
  sfcn : S-Function  InitFcn=rticanmm_initfcn(gcb, 'SFCNs')  FunctionName=RTICANMM_MAIN_CAN_Amk1  SFunctionDeploymentMode=off  EnableBusSupport=off
      mask init:
      | rticanmm_initfcn(gcb, 'SFCNs')
  RX_Data : Outport  VectorParamsAs1DForOutWhenUnconnected=off
  wires:
  Triggering/1 -> rticanmmcycle/1
  rticanmmcycle/1 -> sfcn/1  "<AMK0_ActualValues1_CycleTime>"
  rticanmmcycle/2 -> sfcn/2  "<AMK0_ActualValues2_CycleTime>"
  rticanmmcycle/3 -> sfcn/3  "<AMK0_SetPoints1_CycleTime>"
  rticanmmcycle/4 -> sfcn/4  "<AMK1_ActualValues1_CycleTime>"
  rticanmmcycle/5 -> sfcn/5  "<AMK1_ActualValues2_CycleTime>"
  rticanmmcycle/6 -> sfcn/6  "<AMK1_SetPoints1_CycleTime>"
  TXData/1 -> TXINselector1/1
  TXINselector1/1 -> sfcn/7  "<AMK_bInverterOn>"
  TXINselector1/2 -> sfcn/8  "<AMK_bDcOn>"
  TXINselector1/3 -> sfcn/9  "<AMK_bEnable>"
  TXINselector1/4 -> sfcn/10  "<AMK_bErrorReset>"
  TXINselector1/5 -> sfcn/11  "<AMK_TargetVelocity>"
  TXINselector1/6 -> sfcn/12  "<AMK_TorqueLimitPositiv>"
  TXINselector1/7 -> sfcn/13  "<AMK_TorqueLimitNegativ>"
  TXINselector1/8 -> sfcn/14  "<AMK_bInverterOn>"
  TXINselector1/9 -> sfcn/15  "<AMK_bDcOn>"
  TXINselector1/10 -> sfcn/16  "<AMK_bEnable>"
  TXINselector1/11 -> sfcn/17  "<AMK_bErrorReset>"
  TXINselector1/12 -> sfcn/18  "<AMK_TargetVelocity>"
  TXINselector1/13 -> sfcn/19  "<AMK_TorqueLimitPositiv>"
  TXINselector1/14 -> sfcn/20  "<AMK_TorqueLimitNegativ>"
  converter/1(out) -> RX_Data/1
  sfcn/1 -> converter/1(in_1)
  sfcn/2 -> converter/2(in_2)
  sfcn/3 -> converter/3(in_3)
  sfcn/4 -> converter/4(in_4)
  sfcn/5 -> converter/5(in_5)
  sfcn/6 -> converter/6(in_6)
  sfcn/7 -> converter/7(in_7)
  sfcn/8 -> converter/8(in_8)
  sfcn/9 -> converter/9(in_9)
  sfcn/10 -> converter/10(in_10)
  sfcn/11 -> converter/11(in_11)
  sfcn/12 -> converter/12(in_12)
  sfcn/13 -> converter/13(in_13)
  sfcn/14 -> converter/14(in_14)
  sfcn/15 -> converter/15(in_15)
  sfcn/16 -> converter/16(in_16)
  sfcn/17 -> converter/17(in_17)
  sfcn/18 -> converter/18(in_18)
  sfcn/19 -> converter/19(in_19)
  sfcn/20 -> converter/20(in_20)
  sfcn/21 -> converter/21(in_21)
  sfcn/22 -> converter/22(in_22)
  sfcn/23 -> converter/23(in_23)
  sfcn/24 -> converter/24(in_24)
  sfcn/25 -> converter/25(in_25)
  sfcn/26 -> converter/26(in_26)
  sfcn/27 -> converter/27(in_27)
  sfcn/28 -> converter/28(in_28)
  sfcn/29 -> converter/29(in_29)
  sfcn/30 -> converter/30(in_30)

== system Vcu/Controls /RTICANMM MainBlock1 ==
  TXData : Inport
  ModelClose : Subsystem  mask(RTICANMMModelClose){}
  TRC Exclusion : rtimmsu_dsrtlib/TRC Exclusion
  TXINselector1 : BusSelector  OutputSignals=AMK0_SetPoints1.AMK_bInverterOn,AMK0_SetPoints1.AMK_bDcOn,AMK0_SetPoints1.AMK_bEnable,AMK0_SetPoints1.AMK_bErrorReset,AMK0_SetPoints1.AMK_TargetVelocity,AMK0_SetPoints1.AMK_TorqueLimitPositiv,AMK0_SetPoints1.AMK_TorqueLimitNegativ,AMK1_SetPoints1.AMK_bInverterOn,AMK1_SetPoints1.AMK_bDcOn,AMK1_SetPoints1.AMK_bEnable,AMK1_SetPoints1.AMK_bErrorReset,AMK1_SetPoints1.AMK_TargetVelocity,AMK1_SetPoints1.AMK_TorqueLimitPositiv,AMK1_SetPoints1.AMK_TorqueLimitNegativ
  converter : Subsystem  mask(CANnedyVector2Bus){}
      mask help: Do not change.
      mask Display: disp('Vector to\nBus')
  sfcn : S-Function  InitFcn=rticanmm_initfcn(gcb, 'SFCNs')  FunctionName=RTICANMM_MAIN_CAN_Amk2  SFunctionDeploymentMode=off  EnableBusSupport=off
      mask init:
      | rticanmm_initfcn(gcb, 'SFCNs')
  RX_Data : Outport  VectorParamsAs1DForOutWhenUnconnected=off
  wires:
  TXData/1 -> TXINselector1/1
  TXINselector1/1 -> sfcn/1  "<AMK_bInverterOn>"
  TXINselector1/2 -> sfcn/2  "<AMK_bDcOn>"
  TXINselector1/3 -> sfcn/3  "<AMK_bEnable>"
  TXINselector1/4 -> sfcn/4  "<AMK_bErrorReset>"
  TXINselector1/5 -> sfcn/5  "<AMK_TargetVelocity>"
  TXINselector1/6 -> sfcn/6  "<AMK_TorqueLimitPositiv>"
  TXINselector1/7 -> sfcn/7  "<AMK_TorqueLimitNegativ>"
  TXINselector1/8 -> sfcn/8  "<AMK_bInverterOn>"
  TXINselector1/9 -> sfcn/9  "<AMK_bDcOn>"
  TXINselector1/10 -> sfcn/10  "<AMK_bEnable>"
  TXINselector1/11 -> sfcn/11  "<AMK_bErrorReset>"
  TXINselector1/12 -> sfcn/12  "<AMK_TargetVelocity>"
  TXINselector1/13 -> sfcn/13  "<AMK_TorqueLimitPositiv>"
  TXINselector1/14 -> sfcn/14  "<AMK_TorqueLimitNegativ>"
  converter/1(out) -> RX_Data/1
  sfcn/1 -> converter/1(in_1)
  sfcn/2 -> converter/2(in_2)
  sfcn/3 -> converter/3(in_3)
  sfcn/4 -> converter/4(in_4)
  sfcn/5 -> converter/5(in_5)
  sfcn/6 -> converter/6(in_6)
  sfcn/7 -> converter/7(in_7)
  sfcn/8 -> converter/8(in_8)
  sfcn/9 -> converter/9(in_9)
  sfcn/10 -> converter/10(in_10)
  sfcn/11 -> converter/11(in_11)
  sfcn/12 -> converter/12(in_12)
  sfcn/13 -> converter/13(in_13)
  sfcn/14 -> converter/14(in_14)
  sfcn/15 -> converter/15(in_15)
  sfcn/16 -> converter/16(in_16)
  sfcn/17 -> converter/17(in_17)
  sfcn/18 -> converter/18(in_18)
  sfcn/19 -> converter/19(in_19)
  sfcn/20 -> converter/20(in_20)
  sfcn/21 -> converter/21(in_21)
  sfcn/22 -> converter/22(in_22)
  sfcn/23 -> converter/23(in_23)
  sfcn/24 -> converter/24(in_24)
  sfcn/25 -> converter/25(in_25)
  sfcn/26 -> converter/26(in_26)
  sfcn/27 -> converter/27(in_27)
  sfcn/28 -> converter/28(in_28)
  sfcn/29 -> converter/29(in_29)
  sfcn/30 -> converter/30(in_30)

== system Vcu/Controls /RTICANMM MainBlock2 ==
  TXData : Inport
  ModelClose : Subsystem  mask(RTICANMMModelClose){}
  TRC Exclusion : rtimmsu_dsrtlib/TRC Exclusion
  TXINselector1 : BusSelector  OutputSignals=CoolingLoopModes.InverterLoopFanMode,CoolingLoopModes.InverterLoopPumpMode,CoolingLoopModes.SpeakerRequest,CoolingLoopModes.MotorLoopFanMode,CoolingLoopModes.MotorLoopPumpMode,TemperatureInfo.LeftFrontMotorTemperature,TemperatureInfo.LeftRearMotorTemperature,TemperatureInfo.RightFrontMotorTemperature,TemperatureInfo.RightRearMotorTemperature,TemperatureInfo.BatteryTemperature,VehicleInfo.MaximumPowerAvailablePercentage,VehicleInfo.SocPercentage,VehicleInfo.VcuErrors,VehicleInfo.VehicleSpeed,VehicleInfo.VehicleStatus
  converter : Subsystem  mask(CANnedyVector2Bus){}
      mask help: Do not change.
      mask Display: disp('Vector to\nBus')
  sfcn : S-Function  InitFcn=rticanmm_initfcn(gcb, 'SFCNs')  FunctionName=RTICANMM_MAIN_CAN_Driver  SFunctionDeploymentMode=off  EnableBusSupport=off
      mask init:
      | rticanmm_initfcn(gcb, 'SFCNs')
  RX_Data : Outport  VectorParamsAs1DForOutWhenUnconnected=off
  wires:
  TXData/1 -> TXINselector1/1
  TXINselector1/1 -> sfcn/1  "<InverterLoopFanMode>"
  TXINselector1/2 -> sfcn/2  "<InverterLoopPumpMode>"
  TXINselector1/3 -> sfcn/3  "<SpeakerRequest>"
  TXINselector1/4 -> sfcn/4  "<MotorLoopFanMode>"
  TXINselector1/5 -> sfcn/5  "<MotorLoopPumpMode>"
  TXINselector1/6 -> sfcn/6  "<LeftFrontMotorTemperature>"
  TXINselector1/7 -> sfcn/7  "<LeftRearMotorTemperature>"
  TXINselector1/8 -> sfcn/8  "<RightFrontMotorTemperature>"
  TXINselector1/9 -> sfcn/9  "<RightRearMotorTemperature>"
  TXINselector1/10 -> sfcn/10  "<BatteryTemperature>"
  TXINselector1/11 -> sfcn/11  "<MaximumPowerAvailablePercentage>"
  TXINselector1/12 -> sfcn/12  "<SocPercentage>"
  TXINselector1/13 -> sfcn/13  "<VcuErrors>"
  TXINselector1/14 -> sfcn/14  "<VehicleSpeed>"
  TXINselector1/15 -> sfcn/15  "<VehicleStatus>"
  converter/1(out) -> RX_Data/1
  sfcn/1 -> converter/1(in_1)
  sfcn/2 -> converter/2(in_2)
  sfcn/3 -> converter/3(in_3)
  sfcn/4 -> converter/4(in_4)
  sfcn/5 -> converter/5(in_5)
  sfcn/6 -> converter/6(in_6)
  sfcn/7 -> converter/7(in_7)
  sfcn/8 -> converter/8(in_8)
  sfcn/9 -> converter/9(in_9)
  sfcn/10 -> converter/10(in_10)
  sfcn/11 -> converter/11(in_11)
  sfcn/12 -> converter/12(in_12)
  sfcn/13 -> converter/13(in_13)
  sfcn/14 -> converter/14(in_14)
  sfcn/15 -> converter/15(in_15)
  sfcn/16 -> converter/16(in_16)
  sfcn/17 -> converter/17(in_17)
  sfcn/18 -> converter/18(in_18)
  sfcn/19 -> converter/19(in_19)
  sfcn/20 -> converter/20(in_20)

== system Vcu/Controls /RTICANMM MainBlock3 ==
  TXData : Inport
  ModelClose : Subsystem  mask(RTICANMMModelClose){}
  TRC Exclusion : rtimmsu_dsrtlib/TRC Exclusion
  TXINselector1 : BusSelector  OutputSignals=ELP_ContactorRequest.ELP_Contactor
  converter : Subsystem  mask(CANnedyVector2Bus){}
      mask help: Do not change.
      mask Display: disp('Vector to\nBus')
  sfcn : S-Function  InitFcn=rticanmm_initfcn(gcb, 'SFCNs')  FunctionName=RTICANMM_MAIN_CAN_Ams  SFunctionDeploymentMode=off  EnableBusSupport=off
      mask init:
      | rticanmm_initfcn(gcb, 'SFCNs')
  RX_Data : Outport  VectorParamsAs1DForOutWhenUnconnected=off
  wires:
  TXData/1 -> TXINselector1/1
  TXINselector1/1 -> sfcn/1  "<ELP_Contactor>"
  converter/1(out) -> RX_Data/1
  sfcn/1 -> converter/1(in_1)
  sfcn/2 -> converter/2(in_2)
  sfcn/3 -> converter/3(in_3)
  sfcn/4 -> converter/4(in_4)
  sfcn/5 -> converter/5(in_5)
  sfcn/6 -> converter/6(in_6)
  sfcn/7 -> converter/7(in_7)
  sfcn/8 -> converter/8(in_8)
  sfcn/9 -> converter/9(in_9)
  sfcn/10 -> converter/10(in_10)
  sfcn/11 -> converter/11(in_11)
  sfcn/12 -> converter/12(in_12)
  sfcn/13 -> converter/13(in_13)
  sfcn/14 -> converter/14(in_14)
  sfcn/15 -> converter/15(in_15)
  sfcn/16 -> converter/16(in_16)
  sfcn/17 -> converter/17(in_17)
  sfcn/18 -> converter/18(in_18)
  sfcn/19 -> converter/19(in_19)
  sfcn/20 -> converter/20(in_20)
  sfcn/21 -> converter/21(in_21)
  sfcn/22 -> converter/22(in_22)
  sfcn/23 -> converter/23(in_23)
  sfcn/24 -> converter/24(in_24)
  sfcn/25 -> converter/25(in_25)
  sfcn/26 -> converter/26(in_26)
  sfcn/27 -> converter/27(in_27)
  sfcn/28 -> converter/28(in_28)

== system Vcu/Controls /Signal Builder ==
  Demux : Demux  Tag=STV Demux  Outputs=5
      settings: DisplayOption=none
  FromWs : FromWorkspace  Tag=STV FromWs  VariableName=tuvar
      SigBuilderData=|
      | common.afterFinalStr = 'Extrapolate'
      | common.sampleTime = 0
      | dataSet.timeRange = [0 10]
      | dataSet.name = 'Group 1'
      | sbobj.Groups.Name = 'Group 1'
      | sbobj.Groups.Signals(1).Name = 'AMK_bSystemReady'
      | sbobj.Groups.Signals(1).XData = [0 9.3 9.3 10]
      | sbobj.Groups.Signals(1).YData = [1 1 0 0]
      | sbobj.Groups.Signals(2).Name = 'AMK_bDcOn'
      | sbobj.Groups.Signals(2).XData = [0 0.3 0.3 8.99 8.99 10]
      | sbobj.Groups.Signals(2).YData = [0 0 1 1 0 0]
      | sbobj.Groups.Signals(3).Name = 'AMK_bQuitDcON'
      | sbobj.Groups.Signals(3).XData = [0 0.62 0.62 8.65 8.65 10]
      | sbobj.Groups.Signals(3).YData = [0 0 1 1 0 0]
      | sbobj.Groups.Signals(4).Name = 'AMK_bInverterOn'
      | sbobj.Groups.Signals(4).XData = [0 1 1 8.33 8.33 10]
      | sbobj.Groups.Signals(4).YData = [0 0 1 1 0 0]
      | sbobj.Groups.Signals(5).Name = 'AMK_bQuitInverterOn'
      | sbobj.Groups.Signals(5).XData = [0 1.27 1.27 7.99 7.99 10]
      | sbobj.Groups.Signals(5).YData = [0 0 1 1 0 0]
  AMK_bSystemReady : Outport  Tag=STV Outport  VectorParamsAs1DForOutWhenUnconnected=off
  AMK_bDcOn : Outport  Tag=STV Outport  Port=2  VectorParamsAs1DForOutWhenUnconnected=off
  AMK_bQuitDcON : Outport  Tag=STV Outport  Port=3  VectorParamsAs1DForOutWhenUnconnected=off
  AMK_bInverterOn : Outport  Tag=STV Outport  Port=4  VectorParamsAs1DForOutWhenUnconnected=off
  AMK_bQuitInverterOn : Outport  Tag=STV Outport  Port=5  VectorParamsAs1DForOutWhenUnconnected=off
  wires:
  Demux/1 -> AMK_bSystemReady/1
  Demux/2 -> AMK_bDcOn/1
  Demux/3 -> AMK_bQuitDcON/1
  Demux/4 -> AMK_bInverterOn/1
  Demux/5 -> AMK_bQuitInverterOn/1
  FromWs/1 -> Demux/1

== system Vcu/Controls /Signal Builder1 ==
  Demux : Demux  Tag=STV Demux  Outputs=3
      settings: DisplayOption=none
  FromWs : FromWorkspace  Tag=STV FromWs  VariableName=tuvar
      SigBuilderData=|
      | common.afterFinalStr = 'Extrapolate'
      | common.sampleTime = 0
      | dataSet.timeRange = [0 10]
      | dataSet.name = 'Group 1'
      | sbobj.Groups.Name = 'Group 1'
      | sbobj.Groups.Signals(1).Name = 'K1'
      | sbobj.Groups.Signals(1).XData = [0 0.45 0.45 8 10]
      | sbobj.Groups.Signals(1).YData = [1 1 0 0 0]
      | sbobj.Groups.Signals(2).Name = 'K3'
      | sbobj.Groups.Signals(2).XData = [0 8 8 10]
      | sbobj.Groups.Signals(2).YData = [1 1 0 0]
      | sbobj.Groups.Signals(3).Name = 'K2'
      | sbobj.Groups.Signals(3).XData = [0 0.44 0.44 8 8 10]
      | sbobj.Groups.Signals(3).YData = [0 0 1 1 0 0]
  K1 : Outport  Tag=STV Outport  VectorParamsAs1DForOutWhenUnconnected=off
  K3 : Outport  Tag=STV Outport  Port=2  VectorParamsAs1DForOutWhenUnconnected=off
  K2 : Outport  Tag=STV Outport  Port=3  VectorParamsAs1DForOutWhenUnconnected=off
  wires:
  Demux/1 -> K1/1
  FromWs/1 -> Demux/1
  Demux/2 -> K3/1
  Demux/3 -> K2/1

== system Vcu/Controls /Signal Builder2 ==
  Demux : Demux  Tag=STV Demux  Outputs=5
      settings: DisplayOption=none
  FromWs : FromWorkspace  Tag=STV FromWs  VariableName=tuvar
      SigBuilderData=|
      | common.afterFinalStr = 'Extrapolate'
      | common.sampleTime = 0
      | dataSet.timeRange = [0 10]
      | dataSet.name = 'Group 1'
      | sbobj.Groups.Name = 'Group 1'
      | sbobj.Groups.Signals(1).Name = 'AMK_bSystemReady'
      | sbobj.Groups.Signals(1).XData = [0 9.3 9.3 10]
      | sbobj.Groups.Signals(1).YData = [1 1 0 0]
      | sbobj.Groups.Signals(2).Name = 'AMK_bDcOn'
      | sbobj.Groups.Signals(2).XData = [0 0.3 0.3 8.99 8.99 10]
      | sbobj.Groups.Signals(2).YData = [0 0 1 1 0 0]
      | sbobj.Groups.Signals(3).Name = 'AMK_bQuitDcON'
      | sbobj.Groups.Signals(3).XData = [0 0.62 0.62 8.65 8.65 10]
      | sbobj.Groups.Signals(3).YData = [0 0 1 1 0 0]
      | sbobj.Groups.Signals(4).Name = 'AMK_bInverterOn'
      | sbobj.Groups.Signals(4).XData = [0 1 1 8.33 8.33 10]
      | sbobj.Groups.Signals(4).YData = [0 0 1 1 0 0]
      | sbobj.Groups.Signals(5).Name = 'AMK_bQuitInverterOn'
      | sbobj.Groups.Signals(5).XData = [0 1.27 1.27 7.99 7.99 10]
      | sbobj.Groups.Signals(5).YData = [0 0 1 1 0 0]
  AMK_bSystemReady : Outport  Tag=STV Outport  VectorParamsAs1DForOutWhenUnconnected=off
  AMK_bDcOn : Outport  Tag=STV Outport  Port=2  VectorParamsAs1DForOutWhenUnconnected=off
  AMK_bQuitDcON : Outport  Tag=STV Outport  Port=3  VectorParamsAs1DForOutWhenUnconnected=off
  AMK_bInverterOn : Outport  Tag=STV Outport  Port=4  VectorParamsAs1DForOutWhenUnconnected=off
  AMK_bQuitInverterOn : Outport  Tag=STV Outport  Port=5  VectorParamsAs1DForOutWhenUnconnected=off
  wires:
  Demux/1 -> AMK_bSystemReady/1
  Demux/2 -> AMK_bDcOn/1
  Demux/3 -> AMK_bQuitDcON/1
  Demux/4 -> AMK_bInverterOn/1
  Demux/5 -> AMK_bQuitInverterOn/1
  FromWs/1 -> Demux/1

== system Vcu/Controls /Signal Builder3 ==
  Demux : Demux  Tag=STV Demux  Outputs=5
      settings: DisplayOption=none
  FromWs : FromWorkspace  Tag=STV FromWs  VariableName=tuvar
      SigBuilderData=|
      | common.afterFinalStr = 'Extrapolate'
      | common.sampleTime = 0
      | dataSet.timeRange = [0 10]
      | dataSet.name = 'Group 1'
      | sbobj.Groups.Name = 'Group 1'
      | sbobj.Groups.Signals(1).Name = 'AMK_bSystemReady'
      | sbobj.Groups.Signals(1).XData = [0 9.3 9.3 10]
      | sbobj.Groups.Signals(1).YData = [1 1 0 0]
      | sbobj.Groups.Signals(2).Name = 'AMK_bDcOn'
      | sbobj.Groups.Signals(2).XData = [0 0.3 0.3 8.99 8.99 10]
      | sbobj.Groups.Signals(2).YData = [0 0 1 1 0 0]
      | sbobj.Groups.Signals(3).Name = 'AMK_bQuitDcON'
      | sbobj.Groups.Signals(3).XData = [0 0.62 0.62 8.65 8.65 10]
      | sbobj.Groups.Signals(3).YData = [0 0 1 1 0 0]
      | sbobj.Groups.Signals(4).Name = 'AMK_bInverterOn'
      | sbobj.Groups.Signals(4).XData = [0 1 1 8.33 8.33 10]
      | sbobj.Groups.Signals(4).YData = [0 0 1 1 0 0]
      | sbobj.Groups.Signals(5).Name = 'AMK_bQuitInverterOn'
      | sbobj.Groups.Signals(5).XData = [0 1.27 1.27 7.99 7.99 10]
      | sbobj.Groups.Signals(5).YData = [0 0 1 1 0 0]
  AMK_bSystemReady : Outport  Tag=STV Outport  VectorParamsAs1DForOutWhenUnconnected=off
  AMK_bDcOn : Outport  Tag=STV Outport  Port=2  VectorParamsAs1DForOutWhenUnconnected=off
  AMK_bQuitDcON : Outport  Tag=STV Outport  Port=3  VectorParamsAs1DForOutWhenUnconnected=off
  AMK_bInverterOn : Outport  Tag=STV Outport  Port=4  VectorParamsAs1DForOutWhenUnconnected=off
  AMK_bQuitInverterOn : Outport  Tag=STV Outport  Port=5  VectorParamsAs1DForOutWhenUnconnected=off
  wires:
  Demux/1 -> AMK_bSystemReady/1
  Demux/2 -> AMK_bDcOn/1
  Demux/3 -> AMK_bQuitDcON/1
  Demux/4 -> AMK_bInverterOn/1
  Demux/5 -> AMK_bQuitInverterOn/1
  FromWs/1 -> Demux/1

== system Vcu/Controls /Signal Builder4 ==
  Demux : Demux  Tag=STV Demux  Outputs=5
      settings: DisplayOption=none
  FromWs : FromWorkspace  Tag=STV FromWs  VariableName=tuvar
      SigBuilderData=|
      | common.afterFinalStr = 'Extrapolate'
      | common.sampleTime = 0
      | dataSet.timeRange = [0 10]
      | dataSet.name = 'Group 1'
      | sbobj.Groups.Name = 'Group 1'
      | sbobj.Groups.Signals(1).Name = 'AMK_bSystemReady'
      | sbobj.Groups.Signals(1).XData = [0 9.3 9.3 10]
      | sbobj.Groups.Signals(1).YData = [1 1 0 0]
      | sbobj.Groups.Signals(2).Name = 'AMK_bDcOn'
      | sbobj.Groups.Signals(2).XData = [0 0.3 0.3 8.99 8.99 10]
      | sbobj.Groups.Signals(2).YData = [0 0 1 1 0 0]
      | sbobj.Groups.Signals(3).Name = 'AMK_bQuitDcON'
      | sbobj.Groups.Signals(3).XData = [0 0.62 0.62 8.65 8.65 10]
      | sbobj.Groups.Signals(3).YData = [0 0 1 1 0 0]
      | sbobj.Groups.Signals(4).Name = 'AMK_bInverterOn'
      | sbobj.Groups.Signals(4).XData = [0 1 1 8.33 8.33 10]
      | sbobj.Groups.Signals(4).YData = [0 0 1 1 0 0]
      | sbobj.Groups.Signals(5).Name = 'AMK_bQuitInverterOn'
      | sbobj.Groups.Signals(5).XData = [0 1.27 1.27 7.99 7.99 10]
      | sbobj.Groups.Signals(5).YData = [0 0 1 1 0 0]
  AMK_bSystemReady : Outport  Tag=STV Outport  VectorParamsAs1DForOutWhenUnconnected=off
  AMK_bDcOn : Outport  Tag=STV Outport  Port=2  VectorParamsAs1DForOutWhenUnconnected=off
  AMK_bQuitDcON : Outport  Tag=STV Outport  Port=3  VectorParamsAs1DForOutWhenUnconnected=off
  AMK_bInverterOn : Outport  Tag=STV Outport  Port=4  VectorParamsAs1DForOutWhenUnconnected=off
  AMK_bQuitInverterOn : Outport  Tag=STV Outport  Port=5  VectorParamsAs1DForOutWhenUnconnected=off
  wires:
  Demux/1 -> AMK_bSystemReady/1
  Demux/2 -> AMK_bDcOn/1
  Demux/3 -> AMK_bQuitDcON/1
  Demux/4 -> AMK_bInverterOn/1
  Demux/5 -> AMK_bQuitInverterOn/1
  FromWs/1 -> Demux/1
